simulink model "EvPowertrainController"  (R2017b)
settings: Solver=ode4  StartTime=0.0  StopTime=700  FixedStep=.01  RelTol=1e-3  EnableMultiTasking=on
model workspace (MAT data in the model file):
  Accessory.Power = 1000
  Batt.init_charge = 100
  Batt.Vnom = 320
  Batt.Ah_rating = 100
  Batt.R1 = 0.0846
  Batt.V1 = 283.3
  Batt.Q1 = 10.4
  Batt.Limit.SOC = [0 10 20 30 40 50 60 70 80 90 100]
  Batt.Limit.Discharge = [0 5000 11000 18000 25000 30000 36000 39000 40000 40000 40000]
  Batt.Limit.Charge = [-40000 -40000 -40000 -39000 -36000 -30000 -25000 -18000 -11000 -5000 0]
  Batt.m = 119.7
  Batt.Cp = 101.079756
  CS_SOC_Setpoint = 50
  CS_Thermostat_Off = -5
  CS_Thermostat_On = 0
  CS_Thermostat_Power = [25000 15000 5000 0]
  CS_Thermostat_SOC = [0 50 55 100]
  DCDC.Output_Voltage_Ref = 700
  DCDC.Output_Voltage_Droop = 0.01
  DCDC.Max_Current = 1250
  DCDC.Rated_Output_Power = 400
  DCDC.Efficiency = 96
  DCDC.Fixed_loss = 1e-06
  Diff_ratio = 3.421
  GB_ratio = 2
  OptimPwrVec = Simulink.Parameter
  OptimPwrVec.Value = [2094.39510239 8377.58040957 13351.7687778 19896.7534727 31415.9265359 40840.7044967 56548.6677646 73303.8285838 87964.5943005 95294.9771589]
  OptimPwrVec.DataType = 'auto'
  OptimPwrVec.Dimensions = [1 10]
  OptimSpdVec = Simulink.Parameter
  OptimSpdVec.Value = [500 1000 1500 2000 2500 3000 4000 5000 6000 6500]
  OptimSpdVec.DataType = 'auto'
  OptimSpdVec.Dimensions = [1 10]
  OptimTrqVec = Simulink.Parameter
  OptimTrqVec.Value = [40 80 85 95 120 130 135 140 140 140]
  OptimTrqVec.DataType = 'auto'
  OptimTrqVec.Dimensions = [1 10]
  Pedal.VehSpd_steps = [0 10 20 30 40 50 60 70 80 90 100 110 120 130 140 150 160 170 180]
  Pedal.AccPed_steps = [0 10 20 30 40 50 60 70 80 90 100]
  Pedal.Trq_Scale = [0  10  20  30  40  50  60  70  80  90  100; 0  10  20  30  40  50  60  70  80  90  100; 0  10  20  30  40  50  60  70  80  90  100; 0  10  20  30  40  50  60  70  80  90  100; 0  10  20  30  40  50  60  70  80  90  100; 0  10  20  30  40  50  60  70  80  90  100; 0  10  20  30  40  50  60  70  80  90  100; 0  10  20  30  40  50  60  70  80  90  100; 0  10  20  30  40  50  60  70  80  90  100; 0  10  20  30  40  50  60  70  80  90  100; 0  10  20  30  40  50  60  70  80  90  100; 0  10  20  30  40  50  60  70  80  90  100; 0  10  20  30  40  50  60  70  80  90  100; 0  10  20  30  40  50  60  70  80  90  100; 0  10  20  30  40  50  60  70  80  90  100; 0  10  20  30  40  50  60  70  80  90  100; 0  10  20  30  40  50  60  70  80  90  100; 0  10  20  30  40  50  60  70  80  90  100; 0  10  20  30  40  50  60  70  80  90  100]
  Pedal.Brake_gains = [0.5 0.2 0.2 0.25 0.5 0.5 0.5 0.5 0.5 0.5 0.5 0.5 0.5 0.5 0.5 0.5 0.5 0.5 0.5]
  PowerLimitBuffer = 1500
  SOC.CD_Limit = 80
  SOC.CS_Limit = 50
  mot.max_trq = 120
  mot.max_pwr = 90
  mot.spd = [0 500 1000 1500 2000 2500 3000 3500 7161.97243914 7661.97243914 8161.97243914 8661.97243914 9161.97243914 9661.97243914 10161.9724391 10661.9724391 11161.9724391 11661.9724391 12161.9724391]
  mot.trq = [120 120 120 120 120 120 120 120 120 112.169118269 105.297671501 99.2195136541 93.8047673037 88.9504392721 84.5738066939 80.6076640699 76.9968477689 73.6956545886 70.6658970819]
  mot.map.spdindex = [0 1000 2000 3000 3857 4000 5000 6000 7000 8000 9000 10000 11000 12000 12584]
  mot.map.trqindex = [10 25 50 75 100 125 150 175 200 225 250 275 300 307]
  mot.map.eff = [84  90  90  90  90  90  90  90  90  90  90  90  90  90  90; 84  90  93  95  95  95  96  95  95  95  95  93  93  93  93; 84  90  93  95  95  95  96  95  96  95  95  95  95  93  93; 84  90  93  95  95  95  96  96  96  95  95  95  95  93  93; 84  90  93  95  95  95  96  96  96  95  95  93  93  93  90; 84  88  90  93  93  95  95  96  95  95  95  93  93  93  90; 84  88  90  90  90  93  95  95  95  93  93  93  93  93  90; 84  88  90  90  90  90  93  93  93  93  93  93  93  93  90; 84  84  88  90  90  90  93  93  93  93  93  93  93  93  90; 84  84  88  90  90  90  90  93  93  93  93  93  93  93  90; 84  84  84  90  90  90  90  93  93  93  93  93  93  93  90; 84  84  84  88  90  90  90  93  93  93  93  93  93  93  90; 84  84  84  88  88  88  90  93  93  93  93  93  93  93  90; 84  84  84  88  88  88  90  93  93  93  93  93  93  93  90]
  mot.trq_cp = [120 112.169118269 105.297671501 99.2195136541 93.8047673037 88.9504392721 84.5738066939 80.6076640699 76.9968477689 73.6956545886 70.6658970819 90.4670202838 85.9436692696 81.8511135901 78.1306084269 74.7336254518 71.6197243914 68.7549354157]
  p1 = Simulink.Parameter
  p1.Value = 1.522
  p1.DataType = 'auto'
  p1.Dimensions = [1 1]
  q1 = Simulink.Parameter
  q1.Value = 3.908
  q1.DataType = 'auto'
  q1.Dimensions = [1 1]
  r1 = Simulink.Parameter
  r1.Value = 8137.58744466
  r1.DataType = 'auto'
  r1.Dimensions = [1 1]
  r2 = Simulink.Parameter
  r2.Value = 0
  r2.DataType = 'auto'
  r2.Dimensions = [1 1]
  s1 = Simulink.Parameter
  s1.Value = 20
  s1.DataType = 'auto'
  s1.Dimensions = [1 1]
  s2 = Simulink.Parameter
  s2.Value = 1.6
  s2.DataType = 'auto'
  s2.Dimensions = [1 1]
  tire.rollrad = 0.3
values from neighbouring files (symbols this model uses):
  Batt = 100.0    [EvPowertrainControllerDD.sldd]
  mot = 120.0    [EvPowertrainControllerDD.sldd]
  Pedal : value not decoded    [EvPowertrainControllerDD.sldd]
libraries: simulink x4
settings Model: ModifiedByFormat=The MathWorks, Inc.  Creator=The MathWorks, Inc.  LastModifiedBy=The MathWorks, Inc.
settings DebuggingCC: UnderspecifiedInitializationDetection=Classic  MergeDetectMultiDrivingBlocksExec=none  SFNoUnconditionalDefaultTransitionDiag=warning
settings CodeAppCC: StateflowObjectComments=on
settings GRTTargetCC: TargetLangStandard=C89/C90 (ANSI)
settings ConfigComp: CovMetricSettings=dsw  CovHtmlReporting=on  CovSaveCumulativeToWorkspaceVar=on  CovSaveSingleToWorkspaceVar=on  CovShowResultsExplorer=off  CovExternalEMLEnable=off

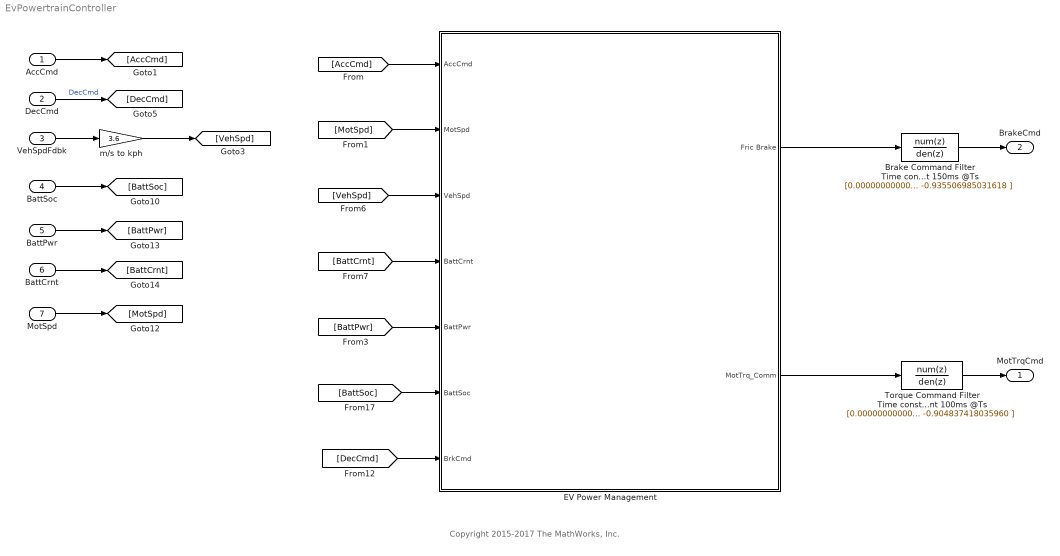
== system EvPowertrainController ==
  note: Copyright 2015-2017 The MathWorks, Inc.
  AccCmd : Inport
  DecCmd : Inport  Port=2  OutDataTypeStr=double
  VehSpdFdbk : Inport  Port=3
  BattSoc : Inport  Port=4
  BattPwr : Inport  Port=5
  BattCrnt : Inport  Port=6
  MotSpd : Inport  Port=7
  Brake Command Filter Time constant 150ms @Ts : DiscreteTransferFcn  Numerator=[0.000000000000000 0.064493014968382 ]  Denominator=[1.000000000000000 -0.935506985031618 ]  SampleTime=0.01  mask(DiscretizedDiscreteTransferFcn){}
      mask init:
      | %zoh
  EV Power Management : Subsystem
  Torque Command Filter Time constant 100ms @Ts : DiscreteTransferFcn  Numerator=[0.000000000000000 0.095162581964040 ]  Denominator=[1.000000000000000 -0.904837418035960 ]  SampleTime=0.01  mask(DiscretizedDiscreteTransferFcn){}
      mask init:
      | %zoh
  m/s to kph : Gain  Gain=3.6
  MotTrqCmd : Outport
  BrakeCmd : Outport  Port=2
  wires:
  EV Power Management/2(MotTrq_Comm) -> Torque Command Filter Time constant 100ms @Ts/1
  VehSpdFdbk/1 -> m/s to kph/1
  [AccCmd] -> EV Power Management/1(AccCmd)
  m/s to kph/1 -> [VehSpd]
  [VehSpd] -> EV Power Management/3(VehSpd)
  DecCmd/1 -> [DecCmd]  "DecCmd"
  [DecCmd] -> EV Power Management/7(BrkCmd)
  BattSoc/1 -> [BattSoc]
  [BattSoc] -> EV Power Management/6(BattSoc)
  [MotSpd] -> EV Power Management/2(MotSpd)
  BattPwr/1 -> [BattPwr]
  [BattPwr] -> EV Power Management/5(BattPwr)
  [BattCrnt] -> EV Power Management/4(BattCrnt)
  BattCrnt/1 -> [BattCrnt]
  AccCmd/1 -> [AccCmd]
  Torque Command Filter Time constant 100ms @Ts/1 -> MotTrqCmd/1
  Brake Command Filter Time constant 150ms @Ts/1 -> BrakeCmd/1
  MotSpd/1 -> [MotSpd]
  EV Power Management/1(Fric Brake) -> Brake Command Filter Time constant 150ms @Ts/1

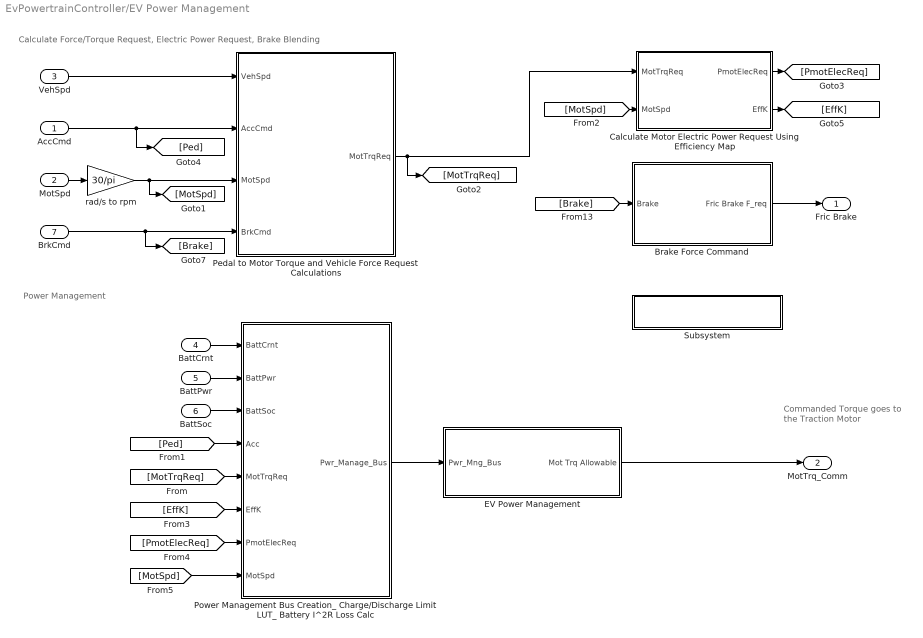
== system EvPowertrainController/EV Power Management ==
  note: Calculate Force/Torque Request, Electric Power Request, Brake Blending
  note: Power Management
  note: Commanded Torque goes to the Traction Motor
  AccCmd : Inport
  MotSpd : Inport  Port=2
  VehSpd : Inport  Port=3
  BattCrnt : Inport  Port=4
  BattPwr : Inport  Port=5
  BattSoc : Inport  Port=6
  BrkCmd : Inport  Port=7
  Brake Force Command : Subsystem
  Calculate Motor Electric Power Request Using Efficiency Map : Subsystem
  EV Power Management : Subsystem
  Pedal to Motor Torque and Vehicle Force Request Calculations : Subsystem
  Power Management Bus Creation_ Charge/Discharge Limit LUT_ Battery I^2R Loss Calc : Subsystem
  Subsystem : Subsystem
      mask Display: fprintf('Power Management Notes')
  rad/s to rpm : Gain  Gain=30/pi
  Fric Brake : Outport
  MotTrq_Comm : Outport  Port=2
  wires:
  Calculate Motor Electric Power Request Using Efficiency Map/1(PmotElecReq) -> [PmotElecReq]
  Power Management Bus Creation_ Charge/Discharge Limit LUT_ Battery I^2R Loss Calc/1(Pwr_Manage_Bus) -> EV Power Management/1(Pwr_Mng_Bus)
  Calculate Motor Electric Power Request Using Efficiency Map/2(EffK) -> [EffK]
  [MotSpd] -> Calculate Motor Electric Power Request Using Efficiency Map/2(MotSpd)
  Pedal to Motor Torque and Vehicle Force Request Calculations/1(MotTrqReq) -> [MotTrqReq], Calculate Motor Electric Power Request Using Efficiency Map/1(MotTrqReq)
  VehSpd/1 -> Pedal to Motor Torque and Vehicle Force Request Calculations/1(VehSpd)
  AccCmd/1 -> Pedal to Motor Torque and Vehicle Force Request Calculations/2(AccCmd), [Ped]
  MotSpd/1 -> rad/s to rpm/1
  BattCrnt/1 -> Power Management Bus Creation_ Charge/Discharge Limit LUT_ Battery I^2R Loss Calc/1(BattCrnt)
  EV Power Management/1(Mot Trq Allowable) -> MotTrq_Comm/1
  BattPwr/1 -> Power Management Bus Creation_ Charge/Discharge Limit LUT_ Battery I^2R Loss Calc/2(BattPwr)
  BattSoc/1 -> Power Management Bus Creation_ Charge/Discharge Limit LUT_ Battery I^2R Loss Calc/3(BattSoc)
  BrkCmd/1 -> [Brake], Pedal to Motor Torque and Vehicle Force Request Calculations/4(BrkCmd)
  [Ped] -> Power Management Bus Creation_ Charge/Discharge Limit LUT_ Battery I^2R Loss Calc/4(Acc)
  [MotTrqReq] -> Power Management Bus Creation_ Charge/Discharge Limit LUT_ Battery I^2R Loss Calc/5(MotTrqReq)
  [EffK] -> Power Management Bus Creation_ Charge/Discharge Limit LUT_ Battery I^2R Loss Calc/6(EffK)
  [PmotElecReq] -> Power Management Bus Creation_ Charge/Discharge Limit LUT_ Battery I^2R Loss Calc/7(PmotElecReq)
  rad/s to rpm/1 -> [MotSpd], Pedal to Motor Torque and Vehicle Force Request Calculations/3(MotSpd)
  [MotSpd] -> Power Management Bus Creation_ Charge/Discharge Limit LUT_ Battery I^2R Loss Calc/8(MotSpd)
  Brake Force Command/1(Fric Brake F_req) -> Fric Brake/1
  [Brake] -> Brake Force Command/1(Brake)

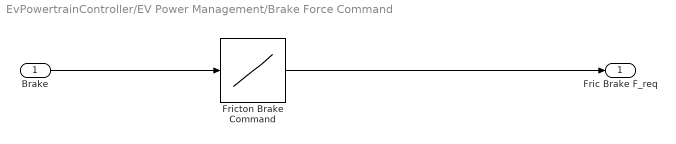
== system EvPowertrainController/EV Power Management/Brake Force Command ==
  Brake : Inport
  Fricton Brake Command : Lookup_n-D  NumberOfTableDimensions=1  BreakpointsForDimension1=[.0 0.1 0.2 0.4 0.6 0.8 1.0]  Table=[0 0 0.2 0.4 0.6 0.8 1.0]*60  ExtrapMethod=Clip  InternalRulePriority=Speed  RndMeth=Simplest  InputSameDT=on
  Fric Brake F_req : Outport
  wires:
  Brake/1 -> Fricton Brake Command/1
  Fricton Brake Command/1 -> Fric Brake F_req/1

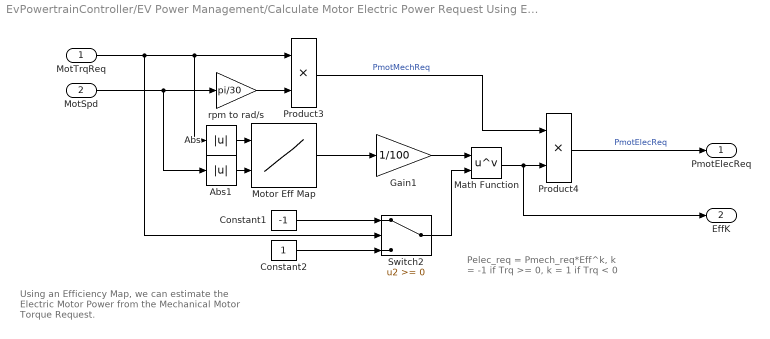
== system EvPowertrainController/EV Power Management/Calculate Motor Electric Power Request Using Efficiency Map ==
  note: Pelec_req = Pmech_req*Eff^k,
      | k = -1 if Trq >= 0,
      | k = 1 if Trq < 0
  note: Using an Efficiency Map, we can estimate the
      | Electric Motor Power from the Mechanical Motor
      | Torque Request.
  MotTrqReq : Inport
  MotSpd : Inport  Port=2
  Abs : Abs
  Abs1 : Abs
  Constant1 : Constant  Value=-1  SampleTime=-1
  Constant2 : Constant  SampleTime=-1
  Gain1 : Gain  Gain=1/100
  Math Function : Math  Operator=pow  OutputSignalType=real  SaturateOnIntegerOverflow=on
  Motor Eff Map : Lookup_n-D  BreakpointsForDimension1=mot.map.trqindex  BreakpointsForDimension2=mot.map.spdindex  Table=mot.map.eff  ExtrapMethod=Clip  UseLastTableValue=on  InternalRulePriority=Speed  OutDataTypeStr=Inherit: Inherit from 'Table data'  RndMeth=Simplest  InputSameDT=on
  Product3 : Product
  Product4 : Product
  Switch2 : Switch
  rpm to rad/s : Gain  Gain=pi/30
  PmotElecReq : Outport
  EffK : Outport  Port=2
  wires:
  Abs1/1 -> Motor Eff Map/2
  Abs/1 -> Motor Eff Map/1
  rpm to rad/s/1 -> Product3/2
  Motor Eff Map/1 -> Gain1/1
  Gain1/1 -> Math Function/1
  Constant2/1 -> Switch2/3
  Constant1/1 -> Switch2/1
  MotTrqReq/1 -> Abs/1, Product3/1, Switch2/2
  Switch2/1 -> Math Function/2
  Product3/1 -> Product4/1  "PmotMechReq"
  MotSpd/1 -> Abs1/1, rpm to rad/s/1
  Product4/1 -> PmotElecReq/1  "PmotElecReq"
  Math Function/1 -> EffK/1, Product4/2

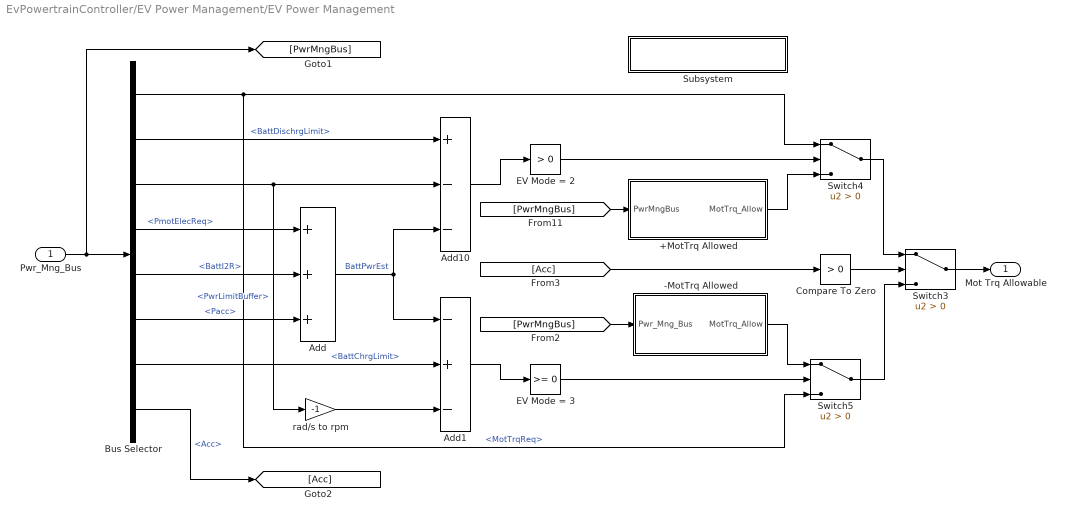
== system EvPowertrainController/EV Power Management/EV Power Management ==
  Pwr_Mng_Bus : Inport
  +MotTrq Allowed : Subsystem
  -MotTrq Allowed : Subsystem
  Add : Sum  Inputs=+++
  Add1 : Sum  Inputs=-+-
  Add10 : Sum  Inputs=+--
  Bus Selector : BusSelector  OutputSignals=MotTrqReq,BattDischrgLimit,PwrLimitBuffer,PmotElecReq,BattI2R,Pacc,BattChrgLimit,Acc
  Compare To Zero : simulink/Logic and Bit Operations/Compare To Zero  relop=>  OutDataTypeStr=boolean
  EV Mode = 2 : simulink/Logic and Bit Operations/Compare To Constant  relop=>  const=0  OutDataTypeStr=boolean
  EV Mode = 3 : simulink/Logic and Bit Operations/Compare To Constant  relop=>=  const=0  OutDataTypeStr=boolean
  Subsystem : Subsystem
      mask Display: fprintf('EV Power Management Notes')
  Switch3 : Switch  Criteria=u2 > Threshold
  Switch4 : Switch  Criteria=u2 > Threshold
  Switch5 : Switch  Criteria=u2 > Threshold
  rad/s to rpm : Gain  Gain=-1
  Mot Trq Allowable : Outport
  wires:
  Compare To Zero/1 -> Switch3/2
  Bus Selector/8 -> [Acc]  "<Acc>"
  [PwrMngBus] -> -MotTrq Allowed/1(Pwr_Mng_Bus)
  Pwr_Mng_Bus/1 -> [PwrMngBus], Bus Selector/1
  [PwrMngBus] -> +MotTrq Allowed/1(PwrMngBus)
  Bus Selector/4 -> Add/1  "<PmotElecReq>"
  Bus Selector/6 -> Add/3  "<Pacc>"
  Bus Selector/5 -> Add/2  "<BattI2R>"
  Add10/1 -> EV Mode = 2/1
  Switch3/1 -> Mot Trq Allowable/1
  rad/s to rpm/1 -> Add1/3
  Bus Selector/3 -> rad/s to rpm/1, Add10/2  "<PwrLimitBuffer>"
  Bus Selector/2 -> Add10/1  "<BattDischrgLimit>"
  Add/1 -> Add1/1, Add10/3  "BattPwrEst"
  Add1/1 -> EV Mode = 3/1
  Bus Selector/7 -> Add1/2  "<BattChrgLimit>"
  Switch4/1 -> Switch3/1
  Switch5/1 -> Switch3/3
  [Acc] -> Compare To Zero/1
  -MotTrq Allowed/1(MotTrq_Allow) -> Switch5/1
  +MotTrq Allowed/1(MotTrq_Allow) -> Switch4/3
  Bus Selector/1 -> Switch4/1, Switch5/3  "<MotTrqReq>"
  EV Mode = 3/1 -> Switch5/2
  EV Mode = 2/1 -> Switch4/2

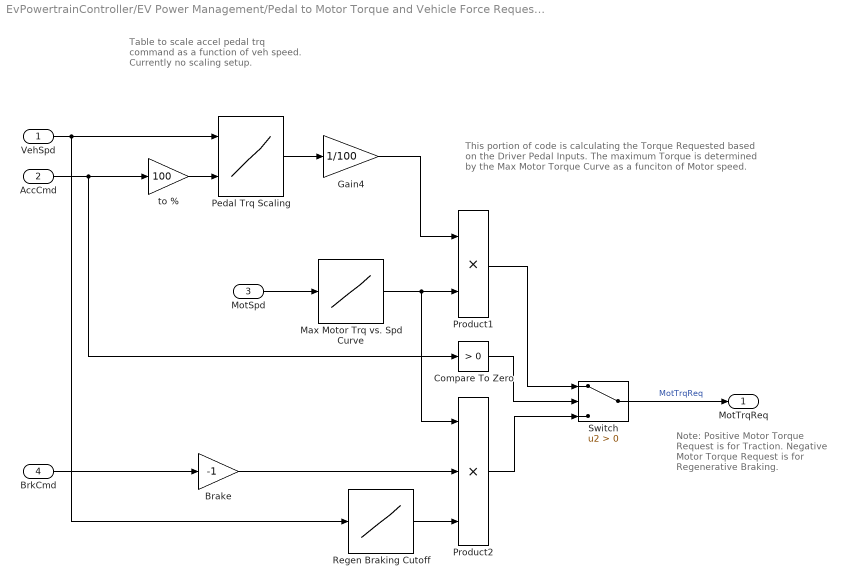
== system EvPowertrainController/EV Power Management/Pedal to Motor Torque and Vehicle Force Request Calculations ==
  note: Table to scale accel pedal trq
      | command as a function of veh
      | speed.  Currently no scaling setup.
  note: This portion of code is calculating the Torque Requested
      | based on the Driver Pedal Inputs.    The maximum Torque
      | is determined by the Max Motor Torque Curve as a funciton
      | of Motor speed.
  note: Note:
      | Positive Motor Torque Request is for Traction.
      | Negative Motor Torque Request is for Regenerative Braking.
  VehSpd : Inport
  AccCmd : Inport  Port=2
  MotSpd : Inport  Port=3
  BrkCmd : Inport  Port=4
  Brake : Gain  Gain=-1
  Compare To Zero : simulink/Logic and Bit Operations/Compare To Zero  relop=>  OutDataTypeStr=boolean
  Gain4 : Gain  Gain=1/100
  Max Motor Trq vs. Spd Curve : Lookup_n-D  NumberOfTableDimensions=1  BreakpointsForDimension1=mot.spd  Table=mot.trq  ExtrapMethod=Clip  UseLastTableValue=on  InternalRulePriority=Speed  OutDataTypeStr=Inherit: Inherit from 'Table data'  RndMeth=Simplest  InputSameDT=on
  Pedal Trq Scaling : Lookup_n-D  BreakpointsForDimension1=Pedal.VehSpd_steps  BreakpointsForDimension2=Pedal.AccPed_steps  Table=Pedal.Trq_Scale  ExtrapMethod=Clip  UseLastTableValue=on  InternalRulePriority=Speed  OutDataTypeStr=Inherit: Inherit from 'Table data'  RndMeth=Simplest  InputSameDT=on
  Product1 : Product
  Product2 : Product  Inputs=3
  Regen Braking Cutoff : Lookup_n-D  NumberOfTableDimensions=1  BreakpointsForDimension1=[0.5 1]  Table=[0 1]  ExtrapMethod=Clip  InternalRulePriority=Speed  RndMeth=Simplest  InputSameDT=on
  Switch : Switch  Criteria=u2 > Threshold
  to % : Gain  Gain=100
  MotTrqReq : Outport
  wires:
  Product1/1 -> Switch/1
  Gain4/1 -> Product1/1
  BrkCmd/1 -> Brake/1
  Pedal Trq Scaling/1 -> Gain4/1
  to %/1 -> Pedal Trq Scaling/2
  Compare To Zero/1 -> Switch/2
  Product2/1 -> Switch/3
  AccCmd/1 -> Compare To Zero/1, to %/1
  Max Motor Trq vs. Spd Curve/1 -> Product1/2, Product2/1
  Switch/1 -> MotTrqReq/1  "MotTrqReq"
  MotSpd/1 -> Max Motor Trq vs. Spd Curve/1
  Brake/1 -> Product2/2
  VehSpd/1 -> Regen Braking Cutoff/1, Pedal Trq Scaling/1
  Regen Braking Cutoff/1 -> Product2/3

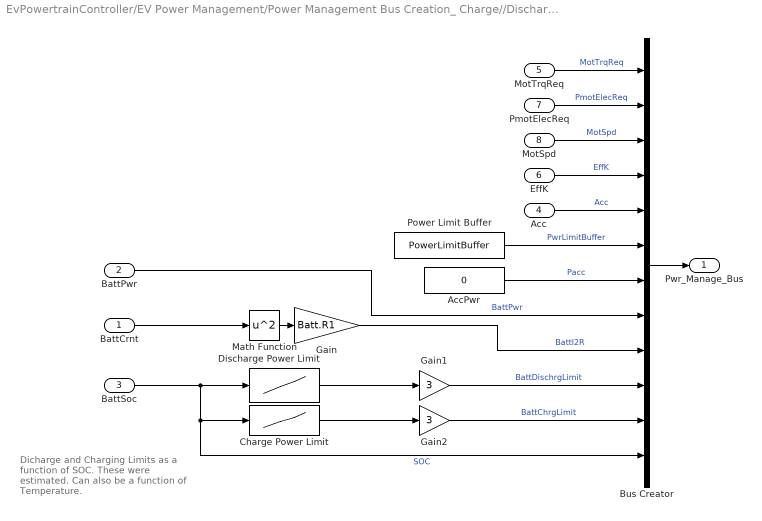
== system EvPowertrainController/EV Power Management/Power Management Bus Creation_ Charge//Discharge Limit LUT_ Battery I^2R Loss Calc ==
  note: Dicharge and Charging Limits as
      | a function of SOC.  These were
      | estimated.  Can also be a function
      | of Temperature.
  BattCrnt : Inport
  BattPwr : Inport  Port=2
  BattSoc : Inport  Port=3
  Acc : Inport  Port=4
  MotTrqReq : Inport  Port=5
  EffK : Inport  Port=6
  PmotElecReq : Inport  Port=7
  MotSpd : Inport  Port=8
  AccPwr : Constant  Value=0
  Bus Creator : BusCreator  Inputs=12
  Charge Power Limit : Lookup_n-D  NumberOfTableDimensions=1  BreakpointsForDimension1=Batt.Limit.SOC  BeginIndexSearchUsingPreviousIndexResult=on  Table=Batt.Limit.Charge  ExtrapMethod=Clip  UseLastTableValue=on  InternalRulePriority=Speed  OutDataTypeStr=Inherit: Inherit from 'Table data'  RndMeth=Simplest  InputSameDT=on
  Discharge Power Limit : Lookup_n-D  NumberOfTableDimensions=1  BreakpointsForDimension1=Batt.Limit.SOC  BeginIndexSearchUsingPreviousIndexResult=on  Table=Batt.Limit.Discharge  ExtrapMethod=Clip  UseLastTableValue=on  InternalRulePriority=Speed  OutDataTypeStr=Inherit: Inherit from 'Table data'  RndMeth=Simplest  InputSameDT=on
  Gain : Gain  Gain=Batt.R1
  Gain1 : Gain  Gain=3
  Gain2 : Gain  Gain=3
  Math Function : Math  Operator=square  SaturateOnIntegerOverflow=on
  Power Limit Buffer : Constant  Value=PowerLimitBuffer
  Pwr_Manage_Bus : Outport
  wires:
  MotTrqReq/1 -> Bus Creator/1  "MotTrqReq"
  Charge Power Limit/1 -> Gain2/1
  Discharge Power Limit/1 -> Gain1/1
  Gain/1 -> Bus Creator/9  "BattI2R"
  PmotElecReq/1 -> Bus Creator/2  "PmotElecReq"
  MotSpd/1 -> Bus Creator/3  "MotSpd"
  AccPwr/1 -> Bus Creator/7  "Pacc"
  EffK/1 -> Bus Creator/4  "EffK"
  Power Limit Buffer/1 -> Bus Creator/6  "PwrLimitBuffer"
  Acc/1 -> Bus Creator/5  "Acc"
  Bus Creator/1 -> Pwr_Manage_Bus/1
  Math Function/1 -> Gain/1
  BattSoc/1 -> Bus Creator/12, Charge Power Limit/1, Discharge Power Limit/1  "SOC"
  BattCrnt/1 -> Math Function/1
  Gain1/1 -> Bus Creator/10  "BattDischrgLimit"
  Gain2/1 -> Bus Creator/11  "BattChrgLimit"
  BattPwr/1 -> Bus Creator/8  "BattPwr"

== system EvPowertrainController/EV Power Management/Subsystem ==
  note: The intent of the EV and HEV Power Management subsystems are to make sure
      | that the Battery Power is not exceeding its Discharge or Charging Limits.

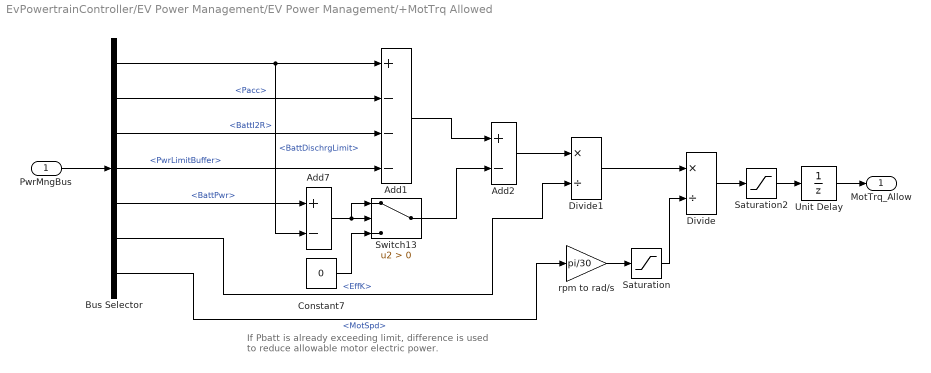
== system EvPowertrainController/EV Power Management/EV Power Management/+MotTrq Allowed ==
  note: If Pbatt is already exceeding limit, difference
      | is used to reduce allowable motor electric power.
  PwrMngBus : Inport
  Add1 : Sum  Inputs=+---
  Add2 : Sum  Inputs=+-
  Add7 : Sum  Inputs=+-
  Bus Selector : BusSelector  OutputSignals=BattDischrgLimit,Pacc,BattI2R,PwrLimitBuffer,BattPwr,EffK,MotSpd
  Constant7 : Constant  Value=0  SampleTime=-1
  Divide : Product  Inputs=*/
  Divide1 : Product  Inputs=*/
  Saturation : Saturate  UpperLimit=inf  LowerLimit=10
  Saturation2 : Saturate  UpperLimit=mot.max_trq  LowerLimit=0
  Switch13 : Switch  Criteria=u2 > Threshold
  Unit Delay : UnitDelay  SampleTime=-1
  rpm to rad/s : Gain  Gain=pi/30
  MotTrq_Allow : Outport
  wires:
  Bus Selector/6 -> Divide1/2  "<EffK>"
  PwrMngBus/1 -> Bus Selector/1
  Unit Delay/1 -> MotTrq_Allow/1
  Add2/1 -> Divide1/1
  Add1/1 -> Add2/1
  Switch13/1 -> Add2/2
  Constant7/1 -> Switch13/3
  Add7/1 -> Switch13/2, Switch13/1
  Bus Selector/5 -> Add7/1  "<BattPwr>"
  Bus Selector/1 -> Add7/2, Add1/1  "<BattDischrgLimit>"
  Bus Selector/4 -> Add1/4  "<PwrLimitBuffer>"
  Bus Selector/3 -> Add1/3  "<BattI2R>"
  Saturation2/1 -> Unit Delay/1
  Divide1/1 -> Divide/1
  Bus Selector/2 -> Add1/2  "<Pacc>"
  Saturation/1 -> Divide/2
  Bus Selector/7 -> rpm to rad/s/1  "<MotSpd>"
  Divide/1 -> Saturation2/1
  rpm to rad/s/1 -> Saturation/1

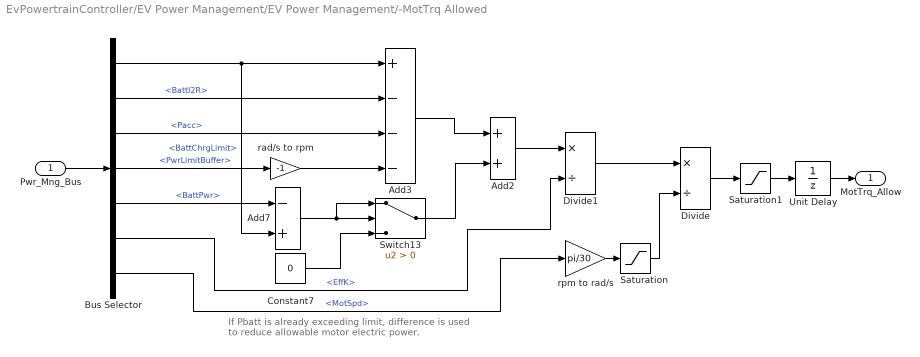
== system EvPowertrainController/EV Power Management/EV Power Management/-MotTrq Allowed ==
  note: If Pbatt is already exceeding limit, difference
      | is used to reduce allowable motor electric power.
  Pwr_Mng_Bus : Inport
  Add2 : Sum
  Add3 : Sum  Inputs=+---
  Add7 : Sum  Inputs=-+
  Bus Selector : BusSelector  OutputSignals=BattChrgLimit,BattI2R,Pacc,PwrLimitBuffer,BattPwr,EffK,MotSpd
  Constant7 : Constant  Value=0  SampleTime=-1
  Divide : Product  Inputs=*/
  Divide1 : Product  Inputs=*/
  Saturation : Saturate  UpperLimit=inf  LowerLimit=10
  Saturation1 : Saturate  UpperLimit=0  LowerLimit=-mot.max_trq
  Switch13 : Switch  Criteria=u2 > Threshold
  Unit Delay : UnitDelay  SampleTime=-1
  rad/s to rpm : Gain  Gain=-1
  rpm to rad/s : Gain  Gain=pi/30
  MotTrq_Allow : Outport
  wires:
  Bus Selector/4 -> rad/s to rpm/1  "<PwrLimitBuffer>"
  Pwr_Mng_Bus/1 -> Bus Selector/1
  Unit Delay/1 -> MotTrq_Allow/1
  rad/s to rpm/1 -> Add3/4
  Bus Selector/5 -> Add7/1  "<BattPwr>"
  Add2/1 -> Divide1/1
  Add3/1 -> Add2/1
  Switch13/1 -> Add2/2
  Constant7/1 -> Switch13/3
  Add7/1 -> Switch13/1, Switch13/2
  Bus Selector/3 -> Add3/3  "<Pacc>"
  Bus Selector/2 -> Add3/2  "<BattI2R>"
  Divide/1 -> Saturation1/1
  Saturation1/1 -> Unit Delay/1
  rpm to rad/s/1 -> Saturation/1
  Bus Selector/7 -> rpm to rad/s/1  "<MotSpd>"
  Saturation/1 -> Divide/2
  Bus Selector/1 -> Add7/2, Add3/1  "<BattChrgLimit>"
  Bus Selector/6 -> Divide1/2  "<EffK>"
  Divide1/1 -> Divide/1

== system EvPowertrainController/EV Power Management/EV Power Management/Subsystem ==
  note: EV Power Management:
      |
      | For EV Power Management, we use a Feed Forward type of Control.
      | 1) Battery Power is Estimated from the Motor Electric Power Request (calculated from Efficiency Map based on Motor Torque Request), Batt I2R losses, and Accessory Power.
      | 2) If Battery Power Estimated + Power Limit Buffer (user defined) is lower than the Battery Power Discharge (or Charge) Limit, then the requested Motor Torque is allowed.
      | 3) If the Battery Power Discharge (or Charge) Limit will be exceeded, then the +/-MotTrq_Allowed Subsystem are used accordingly. The +/-MotTrq_Allowed subsystem uses the Discharge
      | (or Charge) Limit as an upper bound and subtracts the Batt I2R loss, Accessory Power, and Power Limit Buffer, leaving the allowable Motor Electric Power. Using an estimated efficiency
      | and Motor Speed, the estimated allowable Motor Torque is then calcuated (this is the Mechanical Torque that will theoretically not result in the Battery Power to exceed its Limit).
